simulink model "LKAS_AutoSave_DF_20220315_0945"  (R2018b)
settings: Solver=FixedStepDiscrete  StartTime=0.0  StopTime=10.0  FixedStep=0.01  RelTol=1e-3
InitFcn:
  | tmpVer = ver('MATLAB');
  | tmpVer = str2num(tmpVer.Version);
  | % -------------------------------------------------------------------
  | %  MATLAB file generated by Simulink.saveVars on 21-Nov-2019 10:06:14
  | %  MATLAB version: 7.13.0.564 (R2011b)
  | % -------------------------------------------------------------------
  | 
  | 
  | SInt16 = Simulink.AliasType;
  | SInt16.Description = 'Num';
  | if (tmpVer > 7.11)
  | 	SInt16.DataScope = 'Auto';
  | end
  | SInt16.HeaderFile = 'Rte_Type.h';
  | SInt16.BaseType = 'int16';
  | 
  | SInt32 = Simulink.AliasType;
  | SInt32.Description = 'Num';
  | if (tmpVer > 7.11)
  | 	SInt32.DataScope = 'Auto';
  | end
  | SInt32.HeaderFile = 'Rte_Type.h';
  | SInt32.BaseType = 'int32';
  | 
  | SInt8 = Simulink.AliasType;
  | SInt8.Description = 'Num';
  | if (tmpVer > 7.11)
  | 	SInt8.DataScope = 'Auto';
  | end
  | SInt8.HeaderFile = 'Rte_Type.h';
  | SInt8.BaseType = 'int8';
  | 
  | T_A_m2_1024_1_u32 = Simulink.NumericType;
  | T_A_m2_1024_1_u32.Description = 'm2 (square meters  (m2))';
  | if (tmpVer > 7.11)
  | 	T_A_m2_1024_1_u32.DataScope = 'Auto';
  | end
  | T_A_m2_1024_1_u32.HeaderFile = 'Rte_Type.h';
  | T_A_m2_1024_1_u32.DataTypeMode = 'Fixed-point: slope and bias scaling';
  | T_A_m2_1024_1_u32.SignednessBool = false;
  | T_A_m2_1024_1_u32.WordLength = 32;
  | T_A_m2_1024_1_u32.FixedExponent = -10;
  | T_A_m2_1024_1_u32.SlopeAdjustmentFactor = 1;
  | T_A_m2_1024_1_u32.Bias = 0;
  | T_A_m2_1024_1_u32.DataTypeOverride = 'Inherit';
  | T_A_m2_1024_1_u32.IsAlias = true;
  | 
  | T_A_m2_65536_1_u16 = Simulink.NumericType;
  | T_A_m2_65536_1_u16.Description = 'm2 (square meters  (m2))';
  | if (tmpVer > 7.11)
  | 	T_A_m2_65536_1_u16.DataScope = 'Auto';
  | end
  | T_A_m2_65536_1_u16.HeaderFile = 'Rte_Type.h';
  | T_A_m2_65536_1_u16.DataTypeMode = 'Fixed-point: slope and bias scaling';
  | T_A_m2_65536_1_u16.SignednessBool = false;
  | T_A_m2_65536_1_u16.WordLength = 16;
  | T_A_m2_65536_1_u16.FixedExponent = -16;
  | T_A_m2_65536_1_u16.SlopeAdjustmentFactor = 1;
  | T_A_m2_65536_1_u16.Bias = 0;
  | T_A_m2_65536_1_u16.DataTypeOverride = 'Inherit';
  | ... (+4647 lines)
StopFcn:
  | clear  T_A_m2_1024_1_u32 T_A_m2_65536_1_u16 T_A_m2_Float32 T_A_mm2_10_1_u16 T_A_mm2_4_1_s16 T_A_mm2_Float32 T_Cnt_Num_10_1_u32 T_Cnt_Num_1_1_s16 T_Cnt_Num_1_1_s32 T_Cnt_Num_1_1_s8 T_Cnt_Num_1_1_u16 T_Cnt_Num_1_1_u32 T_Cnt_Num_1_1_u8 T_E_J_1_1_s32 T_E_J_Float32 T_E_kJ_128_1_s32 T_E_kJ_Float32 T_E_kwh_10_1_u16 T_E_kwh_Float32 T_Epl_kwhpkm_100_1_u16 T_Epl_kwhpkm_Float32 T_F_N_1_1_s16 T_F_N_Float32 T_I_A_1000_1_u16 T_I_A_1048576_1_s32 T_I_A_2048_1_s16 T_I_A_32_1_s16 T_I_A_Float32 T_I_mA_1_1_s16 T_I_mA_32768_128_s16 T_I_mA_Float32 T_J_kgpm2_128_1_u16 T_J_kgpm2_Float32 T_K_NA_1000_1_s16 T_K_NA_100_1_s16 T_K_NA_100_1_u16 T_K_NA_1024_1_s16 T_K_NA_1024_1_u16 T_K_NA_128_1_s16 T_K_NA_128_1_u16 T_K_NA_128_1_u8 T_K_NA_16777216_1_u32 T_K_NA_16_1_s16 T_K_NA_16_1_u16 T_K_NA_16_1_u8 T_K_NA_1_16_u16 T_K_NA_1_1_s16 T_K_NA_1_1_u16 T_K_NA_1_1_u8 T_K_NA_32768_1_s16 T_K_NA_32768_1_u16 T_K_NA_32_1_s8 T_K_NA_4096_1_u16 T_K_NA_4194304_1_s32 T_K_NA_4194304_1_u16 T_K_NA_65536_1_s32 T_K_NA_65536_1_u16 T_K_NA_8192_1_s16 T_K_NA_8_1_s16 T_K_NA_Float32 T_M_Nm_16_1_s16 T_M_Nm_1_1_s16 T_M_Nm_32768_1_s16 T_M_Nm_32_1_s16 T_M_Nm_4_1_s16 T_M_Nm_512_1_s16 T_M_Nm_Float32 T_P_W_1_4_s16 T_P_W_1_8_s16 T_P_W_Float32 T_P_kW_128_1_s16 T_P_kW_1_8_s16 T_P_kW_8_1_s32 T_P_kW_Float32 T_Pct_pct_1024_1_s32 T_Pct_pct_1024_1_u32 T_Pct_pct_10_1_s16 T_Pct_pct_10_1_u32 T_Pct_pct_128_100_s8 T_Pct_pct_1_1_s16 T_Pct_pct_1_4_u8 T_Pct_pct_255_100_u16 T_Pct_pct_255_100_u8 T_Pct_pct_256_1_s16 T_Pct_pct_256_1_u16 T_Pct_pct_65535_100_u16 T_Pct_pct_Float32 T_R_ohm_1024_1_s16 T_R_ohm_32_1_s16 T_R_ohm_Float32 T_TK_K_16_1_s16 T_TK_K_Float32 T_T_degC_10_400_1_u16 T_T_degC_16_1_s16 T_T_degC_1_40_1_u8 T_T_degC_2_80_1_u8 T_T_degC_Float32 T_U_V_1000_1_u16 T_U_V_10_1_u8 T_U_V_200_1_u8 T_U_V_32_1_s16 T_U_V_4096_1_s16 T_U_V_512_1_s16 T_U_V_65535_8_u16 T_U_V_8192_1_u16 T_U_V_Float32 T_U_mV_1_1_s16 T_U_mV_256_20_u16 T_U_mV_Float32 T_V_l_256_1_s16 T_V_l_4096_1_s16 T_V_l_64_1_s16 T_V_l_65535_100_u16 T_V_l_Float32 T_V_ml_128_1_s16 T_V_ml_1_1_s16 T_V_ml_32768_1_s16 T_V_ml_Float32 T_V_ul_32_1_u16 T_V_ul_Float32 T_Vpl_clpkm_512_1_u16 T_Vpl_clpkm_Float32 T_a_kphps_16_1_s16 T_a_kphps_Float32 T_a_mps2_128_1_s16 T_a_mps2_Float32 T_c_MJpkg_256_1_s16 T_c_MJpkg_Float32 T_c_kJpgpK_1024_1_s16 T_c_kJpgpK_Float32 T_c_kJpkgpK_128_1_u16 T_c_kJpkgpK_Float32 T_chrg_Ah_1_1_s16 T_chrg_Ah_1_1_u16 T_chrg_Ah_1_1_u8 T_chrg_Ah_256_1_u16 T_chrg_Ah_4194304_1_s32 T_chrg_Ah_512_1_u16 T_chrg_Ah_8_1_u16 T_chrg_Ah_Float32 T_cmp_NA_100_1_s16 T_cmp_NA_128_1_s16 T_cmp_NA_16_1_s16 T_cmp_NA_32768_1_u16 T_cmp_NA_Float32 T_d2n_rpmps2_4_1_s16 T_d2n_rpmps2_Float32 T_dPct_pctps_16_1_s16 T_dPct_pctps_256_1_s16 T_dPct_pctps_Float32 T_dT_degCps_128_1_s16 T_dT_degCps_Float32 T_dV_lph_1_1_s16 T_dV_lph_Float32 T_dV_lpm_128_1_s16 T_dV_lpm_32_1_s16 T_dV_lpm_Float32 T_dV_lps_1024_1_u16 T_dV_lps_4_1_u16 T_dV_lps_Float32 T_dV_mlps_1024_1_s16 T_dV_mlps_Float32 T_d_BitField16 T_dm_gps_128_1_s16 T_dm_gps_128_1_u16 T_dm_gps_256_1_u16 T_dm_gps_Float32 T_dm_mgps_1_1_s16 T_dm_mgps_Float32 T_dn_rpmps_1_1_s16 T_dn_rpmps_2_1_s16 T_dn_rpmps_Float32 T_dp_Paps_1_1_s16 T_dp_Paps_Float32 T_dp_kPaps_1_1_s16 T_dp_kPaps_8_1_s16 T_dp_kPaps_Float32 T_dphi_degps_128_1_s16 T_dphi_degps_8_1_s16 T_dphi_degps_Float32 T_dr_ps_256_1_s16 T_dr_ps_Float32 T_drho_mgplps_1_2_s16 T_drho_mgplps_Float32 T_e_NA_1_1_u8 T_f_Hz_1_1_u16 T_f_Hz_1_1_u32 T_f_Hz_64_1_u16 T_f_Hz_8_1_s16 T_f_Hz_Float32 T_g_BitField32 T_l_km_16_1_s16 T_l_km_1_1_u16 T_l_km_1_1_u32 T_l_km_Float32 T_l_m_1024_1_s16 T_l_m_16_1_s16 T_l_m_1_1_u32 T_l_m_Float32 T_l_mm_16_1_s16 T_l_mm_1_1_u16 T_l_mm_4096_1_s16 T_l_mm_4_1_u8 T_l_mm_64_1_s16 T_l_mm_Float32 T_m_g_1_1_s16 T_m_g_2048_1_s16 T_m_g_32_1_u16 T_m_g_Float32 T_m_kg_1024_1_s16 T_m_kg_1_1_s16 T_m_kg_1_1_u32 T_m_kg_Float32 T_m_mg_128_1_s16 T_m_mg_32_1_s16 T_m_mg_Float32 T_n_rpm_1_1_s16 T_n_rpm_1_25_u8 T_n_rpm_256_50_u16 T_n_rpm_2_25_u8 T_n_rpm_4_1_u16 T_n_rpm_Float32 T_p_MPa_64_1_s16 T_p_MPa_Float32 T_p_Pa_1_1_s16 T_p_Pa_Float32 T_p_kPa_1_10_u16 T_p_kPa_1_1_s16 T_p_kPa_1_1_u8 T_p_kPa_256_1_u16 T_p_kPa_32_1_u16 T_p_kPa_64_1_s16 T_p_kPa_Float32 T_phi_deg_100_1_s16 T_phi_deg_1024_1_s16 T_phi_deg_128_1_s16 T_phi_deg_1_1_u8 T_phi_deg_256_1_s16 T_phi_deg_2_1_s8 T_phi_deg_32_1_s16 T_phi_deg_512_6_s32 T_phi_deg_Float32 T_phi_rad_2048_1_s16 T_phi_rad_Float32 T_r_NA_1024_1_s16 T_r_NA_1024_1_u16 T_r_NA_16384_1_s16 T_r_NA_16_1_s16 T_r_NA_256_1_s8 T_r_NA_256_1_u16 T_r_NA_32768_1_u16 T_r_NA_32_1_u16 T_r_NA_4096_1_s16 T_r_NA_65535_2_u16 T_r_NA_8192_1_u16 T_r_NA_Float32 T_rho_gpl_8192_1_s16 T_rho_gpl_Float32 T_rho_kgpm3_16_1_s16 T_rho_kgpm3_Float32 T_rho_mgpl_1_1_s16 T_rho_mgpl_64_1_s16 T_rho_mgpl_Float32 T_t_hour_1_1_s16 T_t_hour_Float32 T_t_m_1_1_u16 T_t_m_Float32 T_t_ms_1_1_s16 T_t_ms_1_1_u16 T_t_ms_1_1_u32 T_t_ms_4096_1_s16 T_t_ms_64_1_s16 T_t_ms_Float32 T_t_s_1000_1_s16 T_t_s_100_1_s16 T_t_s_10_1_s16 T_t_s_10_1_u16 T_t_s_1_1_s16 T_t_s_1_1_u16 T_t_s_1_1_u32 T_t_s_Float32 T_t_us_10_1_u32 T_t_us_1_1_s16 T_t_us_1_1_u32 T_t_us_1_4_u16 T_t_us_Float32 T_v_kph_1_1_u8 T_v_kph_64_1_s16 T_v_kph_64_1_u16 T_v_kph_Float32 T_v_mps_256_1_s16 T_v_mps_Float32 T_w_radps_32_1_s16 T_w_radps_Float32 T_y_BitField8 T_y_BitFieldDiagProgress T_y_BitFieldDiagStatus T_y_NA_1_1_u8 SInt16 SInt32 SInt8 T_BOOLEAN UInt16 UInt32 UInt8 s16 s32 s8 u16 u32 u8
model workspace (MAT data in the model file):
  MCOS : class17 (value not decoded)
  MCOS : class17 (value not decoded)
  MCOS : class17 (value not decoded)
  MCOS : class17 (value not decoded)
  MCOS : class17 (value not decoded)
  MCOS : class17 (value not decoded)
  MCOS : class17 (value not decoded)
  MCOS : class17 (value not decoded)
  MCOS : class17 (value not decoded)
  MCOS : class17 (value not decoded)
  MCOS : class17 (value not decoded)
  MCOS : class17 (value not decoded)
  MCOS : class17 (value not decoded)
  MCOS : class17 (value not decoded)
  MCOS : class17 (value not decoded)
  MCOS : class17 (value not decoded)
  MCOS : class17 (value not decoded)
  MCOS : class17 (value not decoded)
  MCOS : class17 (value not decoded)
  MCOS : class17 (value not decoded)
  MCOS : class17 (value not decoded)
  MCOS : class17 (value not decoded)
  MCOS : class17 (value not decoded)
  MCOS : class17 (value not decoded)
  MCOS : class17 (value not decoded)
  MCOS : class17 (value not decoded)
  MCOS : class17 (value not decoded)
  MCOS : class17 (value not decoded)
  MCOS : class17 (value not decoded)
  MCOS : class17 (value not decoded)
  MCOS : class17 (value not decoded)
  MCOS : class17 (value not decoded)
  MCOS : class17 (value not decoded)
  MCOS : class17 (value not decoded)
  MCOS : class17 (value not decoded)
  MCOS : class17 (value not decoded)
  MCOS : class17 (value not decoded)
  MCOS : class17 (value not decoded)
  MCOS : class17 (value not decoded)
  MCOS : class17 (value not decoded)
  MCOS : class17 (value not decoded)
  MCOS : class17 (value not decoded)
  MCOS : class17 (value not decoded)
  MCOS : class17 (value not decoded)
  MCOS : class17 (value not decoded)
  MCOS : class17 (value not decoded)
  MCOS : class17 (value not decoded)
  MCOS : class17 (value not decoded)
  MCOS : class17 (value not decoded)
  MCOS : class17 (value not decoded)
  MCOS : class17 (value not decoded)
  MCOS : class17 (value not decoded)
  MCOS : class17 (value not decoded)
  MCOS : class17 (value not decoded)
  MCOS : class17 (value not decoded)
  MCOS : class17 (value not decoded)
  MCOS : class17 (value not decoded)
  MCOS : class17 (value not decoded)
  MCOS : class17 (value not decoded)
  MCOS : class17 (value not decoded)
  MCOS : class17 (value not decoded)
  MCOS : class17 (value not decoded)
  MCOS : class17 (value not decoded)
  MCOS : class17 (value not decoded)
  MCOS : class17 (value not decoded)
  MCOS : class17 (value not decoded)
  MCOS : class17 (value not decoded)
  MCOS : class17 (value not decoded)
  MCOS : class17 (value not decoded)
  MCOS : class17 (value not decoded)
  MCOS : class17 (value not decoded)
  MCOS : class17 (value not decoded)
  MCOS : class17 (value not decoded)
  MCOS : class17 (value not decoded)
  MCOS : class17 (value not decoded)
  MCOS : class17 (value not decoded)
  MCOS : class17 (value not decoded)
  MCOS : class17 (value not decoded)
  MCOS : class17 (value not decoded)
  MCOS : class17 (value not decoded)
  MCOS : class17 (value not decoded)
  MCOS : class17 (value not decoded)
  MCOS : class17 (value not decoded)
  MCOS : class17 (value not decoded)
  MCOS : class17 (value not decoded)
  MCOS : class17 (value not decoded)
  MCOS : class17 (value not decoded)
  MCOS : class17 (value not decoded)
  MCOS : class17 (value not decoded)
  MCOS : class17 (value not decoded)
  MCOS : class17 (value not decoded)
  MCOS : class17 (value not decoded)
  MCOS : class17 (value not decoded)
  MCOS : class17 (value not decoded)
  MCOS : class17 (value not decoded)
  MCOS : class17 (value not decoded)
  MCOS : class17 (value not decoded)
  MCOS : class17 (value not decoded)
  MCOS : class17 (value not decoded)
  MCOS : class17 (value not decoded)
  MCOS : class17 (value not decoded)
  MCOS : class17 (value not decoded)
  MCOS : class17 (value not decoded)
  MCOS : class17 (value not decoded)
undefined symbols (not defined in the file): LKA_CarWidth, LKA_SampleTime, LKA_StrRatio_C, LKA_Veh2CamL_C, LKA_Veh2CamW_C, LKA_WhlBaseL_C, LL_CompHdAg_C, LL_CompSWA_C, LL_CrvtPrvwT_C, LL_DesDvt_C, LL_DvtComp_C, LL_DvtPrvwT_C, LL_DvtSpdDet_vDvtSpdMin_C, LL_HandsOff_ExitTime, LL_HandsOff_TextTime, LL_HandsOff_WarnTime, LL_HdAgExT_C, LL_HdAgPrvwT_C, LL_LAccMax_C, LL_LAccRMax_C, LL_LDW_EarliestWarnLine_C, LL_LDW_LatestWarnLine_C, LL_LDWS_SUPPRESS_HEADING, LL_LFClb_TFC_FfCtlRatio_C, LL_LFClb_TFC_KdBalance_C, LL_LFClb_TFC_KdMaxSWA_C, LL_LFClb_TFC_KdV1_C, LL_LFClb_TFC_KdV2_C, LL_LFClb_TFC_KdVehSpdLwr_C, LL_LFClb_TFC_KdVehSpdUpr_C, LL_LFClb_TFC_Ki_C, LL_LFClb_TFC_KiMaxSWA_C, LL_LFClb_TFC_Kp_C, LL_LFClb_TFC_KpKlat_C, LL_LFClb_TFC_KpV1_C, LL_LFClb_TFC_KpV2_C, LL_LFClb_TFC_KpVehSpdLwr_C, LL_LFClb_TFC_KpVehSpdUpr_C, LL_LFClb_TFC_PrvwT_C, LL_LKA_EarliestWarnLine_C, LL_LKA_LatestWarnLine_C, LL_LKAExPrcs_ExitC0Dvt, LL_LKAExPrcs_ExitC0Swt, LL_LKAExPrcs_tiExitDelayTime3, LL_LKAExPrcs_tiExitTime1, LL_LKAExPrcs_tiExitTime2, LL_LKAExPrcs_tiExitTime3, LL_LKAS_OUT_OF_CONTROL_LAT_VEL, LL_LKAS_OUT_OF_CONTROL_TTLC, LL_LKASWASyn_M0, LL_LKASWASyn_M1, LL_LKASWASyn_M2, LL_LKASWASyn_M3D, LL_LKASWASyn_M3K, LL_LKASWASyn_SWAaddMax, LL_LKASWASyn_T2, LL_LKASWASyn_tiTrqSwaRtTime, LL_LKASWASyn_tiTrqSwaTime, LL_LKASWASyn_TrqMax, LL_LKASWASyn_TrqSwaAddSwt ... (+45)
libraries: simulink x139, canmsglib x8, dspstat3 x3, simulink_extras x1
(part 18 of 20)

== system LKAS_AutoSave_DF_20220315_0945/LKAS/LL/LLOn/LL State Determination (LLStateDet)/LL State Machine Conditions (LLSMCon)/Deactivation Condition (DeactvC)/Deviation Threshold Condition (DvtThresCon)/Deviation Threshold Judgement LDW (DvtThresJdg)/Deviation Threshold Condition Synthesis (DTCSyn) ==
  note: 累计激活LDW的时间，报警时间超过2s触发Deactive;
      | 检测到上升沿，即从离开报警区域，到再次进入报警区域，触发Activeflg，重新计时。
  DTCSyn_stLftDvtThresActvFlg : Inport
  DTCSyn_stRgtDvtThresActvFlg : Inport  Port=2
  DTCSyn_stDvtSpdFlg : Inport  Port=3
  SampleTime : Inport  Port=4
  Bus Selector1 : BusSelector  OutputSignals=bsConstantClb.LKA_SampleTime
  Cast To Single{,1,3..4} (4 alike) : DataTypeConversion  OutDataTypeStr=uint8
  Cast To Single2 : DataTypeConversion  LockScale=on
  Constant : Constant  Value=2  OutDataTypeStr=single
  Constant2 : Constant  Value=0  OutDataTypeStr=uint8
  Divide : Product  Inputs=**  OutDataTypeStr=uint8
  Gain1 : Gain  Gain=2  OutDataTypeStr=Inherit: Same as input
  Sum Condition : Subsystem
  Switch2 : Switch  Criteria=u2 > Threshold
  Switch3 : Switch
  DTCSyn_stDvtThresActvFlg : Outport
  wires:
  Cast To Single1/1 -> Gain1/1
  Cast To Single/1 -> Cast To Single2/1
  Gain1/1 -> Switch3/3  "DvtThresActvFlg"
  Cast To Single2/1 -> Switch2/1  "DvtThresActvFlg"
  Constant2/1 -> Switch2/3  "DvtThresActvFlg"
  DTCSyn_stDvtSpdFlg/1 -> Switch2/2, Switch3/2
  Switch2/1 -> Switch3/1
  DTCSyn_stLftDvtThresActvFlg/1 -> Cast To Single/1
  DTCSyn_stRgtDvtThresActvFlg/1 -> Cast To Single1/1
  Bus Selector1/1 -> Sum Condition/1(In)  "<LKA_SampleTime>"
  Constant/1 -> Sum Condition/2(Sum)
  SampleTime/1 -> Bus Selector1/1
  Switch3/1 -> Cast To Single3/1, Sum Condition/Enable
  Sum Condition/1(Out) -> Cast To Single4/1
  Divide/1 -> DTCSyn_stDvtThresActvFlg/1
  Cast To Single3/1 -> Divide/1
  Cast To Single4/1 -> Divide/2

== system LKAS_AutoSave_DF_20220315_0945/LKAS/LL/LLOn/LL State Determination (LLStateDet)/LL State Machine Conditions (LLSMCon)/Deactivation Condition (DeactvC)/Deviation Threshold Condition (DvtThresCon)/Deviation Threshold Judgement LDW (DvtThresJdg)/Left Side Deviation Threshold Condition (LftDTC) ==
  LftDTC_bsDvtThresInfo : Inport
  LftDTC_lLftDvt : Inport  Port=2
  LftDTC_vLftDvtSpd : Inport  Port=3
  Abs : Abs
  Bus Selector : BusSelector  OutputSignals=LL_ThresDet_lDvtThresLwrLDW,LL_ThresDet_lDvtThresUprLDW,LL_ThresDet_tiTTLCThresLDW
  Divide : Product  Inputs=**
  Relational Operator2 : RelationalOperator  Operator=<=  OutDataTypeStr=boolean  RndMeth=Nearest
  Saturation Dynamic : simulink/Discontinuities/Saturation Dynamic  OutMin=[]  OutMax=[]  OutDataTypeStr=Inherit: Same as second input  OutDataType=fixdt(1, 16)  OutScaling=2^-10  DoSatur=off
  LftDTC_stLftDvtThresActvFlg : Outport
  wires:
  Abs/1 -> Divide/2
  Saturation Dynamic/1 -> Relational Operator2/2
  Divide/1 -> Saturation Dynamic/2
  LftDTC_vLftDvtSpd/1 -> Abs/1
  LftDTC_lLftDvt/1 -> Relational Operator2/1
  Relational Operator2/1 -> LftDTC_stLftDvtThresActvFlg/1
  Bus Selector/2 -> Saturation Dynamic/1  "<LL_ThresDet_lDvtThresUprLDW>"
  Bus Selector/3 -> Divide/1  "<LL_ThresDet_tiTTLCThresLDW>"
  Bus Selector/1 -> Saturation Dynamic/3  "<LL_ThresDet_lDvtThresLwrLDW>"
  LftDTC_bsDvtThresInfo/1 -> Bus Selector/1

== system LKAS_AutoSave_DF_20220315_0945/LKAS/LL/LLOn/LL State Determination (LLStateDet)/LL State Machine Conditions (LLSMCon)/Deactivation Condition (DeactvC)/Deviation Threshold Condition (DvtThresCon)/Deviation Threshold Judgement LDW (DvtThresJdg)/Right Side Deviation Threshold Condition (RgtDTC) ==
  RgtDTC_bsDvtThresInfo : Inport
  RgtDTC_lRgtDvt : Inport  Port=2
  RgtDTC_vRgtDvtSpd : Inport  Port=3
  Abs : Abs
  Bus Selector : BusSelector  OutputSignals=LL_ThresDet_lDvtThresLwrLDW,LL_ThresDet_lDvtThresUprLDW,LL_ThresDet_tiTTLCThresLDW
  Divide : Product  Inputs=**
  Relational Operator2 : RelationalOperator  Operator=<=  OutDataTypeStr=boolean  RndMeth=Nearest
  Saturation Dynamic : simulink/Discontinuities/Saturation Dynamic  OutMin=[]  OutMax=[]  OutDataTypeStr=Inherit: Same as second input  OutDataType=fixdt(1, 16)  OutScaling=2^-10  DoSatur=off
  RgtDTC_stRgtDvtThresActvFlg : Outport
  wires:
  Bus Selector/3 -> Divide/1  "<LL_ThresDet_tiTTLCThresLDW>"
  Bus Selector/2 -> Saturation Dynamic/1  "<LL_ThresDet_lDvtThresUprLDW>"
  Bus Selector/1 -> Saturation Dynamic/3  "<LL_ThresDet_lDvtThresLwrLDW>"
  RgtDTC_vRgtDvtSpd/1 -> Abs/1
  Saturation Dynamic/1 -> Relational Operator2/2
  Divide/1 -> Saturation Dynamic/2
  Abs/1 -> Divide/2
  RgtDTC_lRgtDvt/1 -> Relational Operator2/1
  Relational Operator2/1 -> RgtDTC_stRgtDvtThresActvFlg/1
  RgtDTC_bsDvtThresInfo/1 -> Bus Selector/1

== system LKAS_AutoSave_DF_20220315_0945/LKAS/LL/LLOn/LL State Determination (LLStateDet)/LL State Machine Conditions (LLSMCon)/Deactivation Condition (DeactvC)/Deviation Threshold Condition (DvtThresCon)/Deviation Threshold Judgement LKA (DvtThresJdg)/Deviation Speed Detection (DvtSpdDet) ==
  DvtSpdDet_vLftDvtSpd : Inport
  DvtSpdDet_vRgtDvtSpd : Inport  Port=2
  DvtSpdDet_vDvtSpdMin_C : Inport  Port=3
  If : If  NumInputs=3  IfExpression=u1>=u3 | u2>=u3  ElseIfExpressions=u1<=-u3 | u2<=-u3
  Merge1 : Merge  Inputs=3
  Ph1SWA : Subsystem
  Ph2SWA : Subsystem
  Ph3SWA : Subsystem
  DvtSpdDet_stDvtSpdFlg : Outport
  wires:
  DvtSpdDet_vLftDvtSpd/1 -> If/1
  DvtSpdDet_vRgtDvtSpd/1 -> If/2
  DvtSpdDet_vDvtSpdMin_C/1 -> If/3
  If/1 -> Ph1SWA/Action
  Ph1SWA/1(Out) -> Merge1/1
  Ph2SWA/1(Out) -> Merge1/2
  Ph3SWA/1(Out) -> Merge1/3
  If/2 -> Ph2SWA/Action
  If/3 -> Ph3SWA/Action
  Merge1/1 -> DvtSpdDet_stDvtSpdFlg/1

== system LKAS_AutoSave_DF_20220315_0945/LKAS/LL/LLOn/LL State Determination (LLStateDet)/LL State Machine Conditions (LLSMCon)/Deactivation Condition (DeactvC)/Deviation Threshold Condition (DvtThresCon)/Deviation Threshold Judgement LKA (DvtThresJdg)/Deviation Threshold Condition Synthesis (DTCSyn) ==
  DTCSyn_stLftDvtThresActvFlg : Inport
  DTCSyn_stRgtDvtThresActvFlg : Inport  Port=2
  DTCSyn_stDvtSpdFlg : Inport  Port=3
  Cast To Single : DataTypeConversion  OutDataTypeStr=uint8
  Cast To Single1 : DataTypeConversion  OutDataTypeStr=uint8
  Cast To Single2 : DataTypeConversion  LockScale=on
  Constant2 : Constant  Value=0  OutDataTypeStr=uint8
  Gain1 : Gain  Gain=2  OutDataTypeStr=Inherit: Same as input
  Switch2 : Switch  Criteria=u2 > Threshold
  Switch3 : Switch
  DTCSyn_stDvtThresActvFlg : Outport
  wires:
  Cast To Single1/1 -> Gain1/1
  Cast To Single/1 -> Cast To Single2/1
  Switch2/1 -> Switch3/1
  Switch3/1 -> DTCSyn_stDvtThresActvFlg/1
  Constant2/1 -> Switch2/3  "DvtThresActvFlg"
  DTCSyn_stDvtSpdFlg/1 -> Switch2/2, Switch3/2
  Cast To Single2/1 -> Switch2/1  "DvtThresActvFlg"
  Gain1/1 -> Switch3/3  "DvtThresActvFlg"
  DTCSyn_stLftDvtThresActvFlg/1 -> Cast To Single/1
  DTCSyn_stRgtDvtThresActvFlg/1 -> Cast To Single1/1

== system LKAS_AutoSave_DF_20220315_0945/LKAS/LL/LLOn/LL State Determination (LLStateDet)/LL State Machine Conditions (LLSMCon)/Deactivation Condition (DeactvC)/Deviation Threshold Condition (DvtThresCon)/Deviation Threshold Judgement LKA (DvtThresJdg)/Left Side Deviation Threshold Condition (LftDTC) ==
  LftDTC_bsDvtThresInfo : Inport
  LftDTC_lLftDvt : Inport  Port=2
  LftDTC_vLftDvtSpd : Inport  Port=3
  Abs : Abs
  Bus Selector : BusSelector  OutputSignals=LL_ThresDet_lDvtThresLwrLKA,LL_ThresDet_lDvtThresUprLKA,LL_ThresDet_tiTTLCThresLKA
  Constant : Constant  Value=0  OutDataTypeStr=single
  Divide : Product  Inputs=**
  Logical Operator : Logic  AllPortsSameDT=off  OutDataTypeStr=boolean
  Relational Operator1 : RelationalOperator  Operator=<  OutDataTypeStr=boolean  RndMeth=Nearest
  Relational Operator3 : RelationalOperator  Operator=<=  OutDataTypeStr=boolean  RndMeth=Nearest
  Saturation Dynamic : simulink/Discontinuities/Saturation Dynamic  OutMin=[]  OutMax=[]  OutDataTypeStr=Inherit: Same as second input  OutDataType=fixdt(1, 16)  OutScaling=2^-10  DoSatur=off
  LftDTC_stLftDvtThresActvFlg : Outport
  wires:
  LftDTC_bsDvtThresInfo/1 -> Bus Selector/1
  Bus Selector/1 -> Saturation Dynamic/3  "<LL_ThresDet_lDvtThresLwrLKA>"
  Bus Selector/3 -> Divide/1  "<LL_ThresDet_tiTTLCThresLKA>"
  Bus Selector/2 -> Saturation Dynamic/1  "<LL_ThresDet_lDvtThresUprLKA>"
  Relational Operator3/1 -> Logical Operator/2
  LftDTC_lLftDvt/1 -> Relational Operator1/2, Relational Operator3/1
  LftDTC_vLftDvtSpd/1 -> Abs/1
  Divide/1 -> Saturation Dynamic/2
  Saturation Dynamic/1 -> Relational Operator3/2
  Abs/1 -> Divide/2
  Logical Operator/1 -> LftDTC_stLftDvtThresActvFlg/1
  Constant/1 -> Relational Operator1/1
  Relational Operator1/1 -> Logical Operator/1

== system LKAS_AutoSave_DF_20220315_0945/LKAS/LL/LLOn/LL State Determination (LLStateDet)/LL State Machine Conditions (LLSMCon)/Deactivation Condition (DeactvC)/Deviation Threshold Condition (DvtThresCon)/Deviation Threshold Judgement LKA (DvtThresJdg)/Right Side Deviation Threshold Condition (RgtDTC) ==
  RgtDTC_bsDvtThresInfo : Inport
  RgtDTC_lRgtDvt : Inport  Port=2
  RgtDTC_vRgtDvtSpd : Inport  Port=3
  Abs : Abs
  Bus Selector : BusSelector  OutputSignals=LL_ThresDet_lDvtThresLwrLKA,LL_ThresDet_lDvtThresUprLKA,LL_ThresDet_tiTTLCThresLKA
  Constant : Constant  Value=0  OutDataTypeStr=single
  Divide : Product  Inputs=**
  Logical Operator : Logic  AllPortsSameDT=off  OutDataTypeStr=boolean
  Relational Operator1 : RelationalOperator  Operator=<  OutDataTypeStr=boolean  RndMeth=Nearest
  Relational Operator2 : RelationalOperator  Operator=<=  OutDataTypeStr=boolean  RndMeth=Nearest
  Saturation Dynamic : simulink/Discontinuities/Saturation Dynamic  OutMin=[]  OutMax=[]  OutDataTypeStr=Inherit: Same as second input  OutDataType=fixdt(1, 16)  OutScaling=2^-10  DoSatur=off
  RgtDTC_stRgtDvtThresActvFlg : Outport
  wires:
  Abs/1 -> Divide/2
  RgtDTC_bsDvtThresInfo/1 -> Bus Selector/1
  Relational Operator2/1 -> Logical Operator/2
  RgtDTC_vRgtDvtSpd/1 -> Abs/1
  Divide/1 -> Saturation Dynamic/2
  Saturation Dynamic/1 -> Relational Operator2/2
  Bus Selector/1 -> Saturation Dynamic/3  "<LL_ThresDet_lDvtThresLwrLKA>"
  Bus Selector/2 -> Saturation Dynamic/1  "<LL_ThresDet_lDvtThresUprLKA>"
  Bus Selector/3 -> Divide/1  "<LL_ThresDet_tiTTLCThresLKA>"
  Constant/1 -> Relational Operator1/1
  Relational Operator1/1 -> Logical Operator/1
  RgtDTC_lRgtDvt/1 -> Relational Operator1/2, Relational Operator2/1
  Logical Operator/1 -> RgtDTC_stRgtDvtThresActvFlg/1

== system LKAS_AutoSave_DF_20220315_0945/LKAS/LL/LLOn/LL State Determination (LLStateDet)/LL State Machine Conditions (LLSMCon)/Deactivation Condition (DeactvC)/Driver Take Condition (DvrTkCon)/Time Delay (TDel)/If Action Subsystem ==
  Action Port : ActionPort  InitializeStates=reset  ActionType=then
      settings: AttributesFormatString=states = %<InitializeStates>
  Constant : Constant  OutDataTypeStr=boolean  SampleTime=-1
  Out : Outport
      settings: AttributesFormatString=%<OutputWhenDisabled> = %<InitialOutput>
  wires:
  Constant/1 -> Out/1

== system LKAS_AutoSave_DF_20220315_0945/LKAS/LL/LLOn/LL State Determination (LLStateDet)/LL State Machine Conditions (LLSMCon)/Deactivation Condition (DeactvC)/Driver Take Condition (DvrTkCon)/Time Delay (TDel)/If Action Subsystem1 ==
  Action Port : ActionPort  InitializeStates=reset  ActionType=elseif
      settings: AttributesFormatString=states = %<InitializeStates>
  Constant : Constant  Value=0  OutDataTypeStr=boolean  SampleTime=-1
  Out : Outport
      settings: AttributesFormatString=%<OutputWhenDisabled> = %<InitialOutput>
  wires:
  Constant/1 -> Out/1

== system LKAS_AutoSave_DF_20220315_0945/LKAS/LL/LLOn/LL State Determination (LLStateDet)/LL State Machine Conditions (LLSMCon)/Deactivation Condition (DeactvC)/Driver Take Condition (DvrTkCon)/Time Delay (TDel)/If Action Subsystem3 ==
  In1 : Inport
  Action Port : ActionPort  InitializeStates=reset  ActionType=else
      settings: AttributesFormatString=states = %<InitializeStates>
  Out : Outport
      settings: AttributesFormatString=%<OutputWhenDisabled> = %<InitialOutput>
  wires:
  In1/1 -> Out/1

== system LKAS_AutoSave_DF_20220315_0945/LKAS/LL/LLOn/LL State Determination (LLStateDet)/LL State Machine Conditions (LLSMCon)/Deactivation Condition (DeactvC)/Driver Take Condition (DvrTkCon)/Time Delay (TDel)/Sum Condition1 ==
  SampleTime : Inport
  Sum : Inport  Port=2
  state = reset : EnablePort  StatesWhenEnabling=reset
  Add1 : Sum  OutDataTypeStr=single
  Memory : Memory  InheritSampleTime=on
  Relational Operator : RelationalOperator  Operator=<=  OutDataTypeStr=boolean  RndMeth=Nearest
  Saturation : Saturate  UpperLimit=5  LowerLimit=0
      settings: AttributesFormatString="Min = %<LowerLimit>  Max = %<UpperLimit>"
  Out : Outport  OutputWhenDisabled=reset  InitialOutput=0
      settings: AttributesFormatString=%<OutputWhenDisabled> = %<InitialOutput>
  wires:
  Memory/1 -> Add1/2
  Add1/1 -> Saturation/1
  SampleTime/1 -> Add1/1
  Sum/1 -> Relational Operator/2
  Relational Operator/1 -> Out/1
  Saturation/1 -> Memory/1, Relational Operator/1

== system LKAS_AutoSave_DF_20220315_0945/LKAS/LL/LLOn/LL State Determination (LLStateDet)/LL State Machine Conditions (LLSMCon)/Disable Condition (DisblC)/Driver Intent Condition (DrvInttC)/Driver Release Detection (DrvRlsDet)/ExitCount ==
  SampleTime : Inport
  ExitTime : Inport  Port=2
  Enable : EnablePort  StatesWhenEnabling=reset
  Add : Sum  OutDataTypeStr=single
  Memory : Memory  InheritSampleTime=on
  Relational Operator : RelationalOperator  OutDataTypeStr=boolean  RndMeth=Nearest
  Saturation : Saturate  UpperLimit=60  LowerLimit=0
      settings: AttributesFormatString="Min = %<LowerLimit>  Max = %<UpperLimit>"
  Out : Outport  OutputWhenDisabled=reset  InitialOutput=0
      settings: AttributesFormatString=%<OutputWhenDisabled> = %<InitialOutput>
  wires:
  Memory/1 -> Add/2
  Saturation/1 -> Relational Operator/1, Memory/1
  Add/1 -> Saturation/1
  Relational Operator/1 -> Out/1
  SampleTime/1 -> Add/1
  ExitTime/1 -> Relational Operator/2

== system LKAS_AutoSave_DF_20220315_0945/LKAS/LL/LLOn/LL State Determination (LLStateDet)/LL State Machine Conditions (LLSMCon)/Disable Condition (DisblC)/Driver Intent Condition (DrvInttC)/Take-Over Steering Check (TkOvStChk)/Sum Condition1 ==
  In : Inport
  Sum : Inport  Port=2
  state = reset : EnablePort  StatesWhenEnabling=reset
  Add1 : Sum  AccumDataTypeStr=single  OutDataTypeStr=single
  Memory : Memory  InheritSampleTime=on
  Relational Operator : RelationalOperator  OutDataTypeStr=boolean  RndMeth=Nearest
  Saturation : Saturate  UpperLimit=5000  LowerLimit=0
      settings: AttributesFormatString="Min = %<LowerLimit>  Max = %<UpperLimit>"
  Out : Outport  OutputWhenDisabled=reset  InitialOutput=0
      settings: AttributesFormatString=%<OutputWhenDisabled> = %<InitialOutput>
  wires:
  Memory/1 -> Add1/2
  Add1/1 -> Saturation/1
  In/1 -> Add1/1
  Sum/1 -> Relational Operator/2
  Relational Operator/1 -> Out/1
  Saturation/1 -> Memory/1, Relational Operator/1

== system LKAS_AutoSave_DF_20220315_0945/LKAS/LL/LLOn/LL State Determination (LLStateDet)/LL State Machine Conditions (LLSMCon)/Disable Condition (DisblC)/Driver Intent Condition (DrvInttC)/Take-Over Steering Check (TkOvStChk)/Time Delay (TDel) ==
  TDel_stFlgIn : Inport
  SampleTime : Inport  Port=2
  TDel_tiTDel : Inport  Port=3
  Detect Rise Positive : simulink/Logic and Bit Operations/Detect Rise Positive  vinit=0  OutDataTypeStr=boolean
  If : If  IfExpression=u1
  If Action Subsystem : Subsystem  TreatAsAtomicUnit=on
  If Action Subsystem3 : Subsystem  TreatAsAtomicUnit=on
  Logical Operator : Logic  Operator=OR  AllPortsSameDT=off  OutDataTypeStr=boolean
  Merge : Merge
  Sum Condition1 : Subsystem  TreatAsAtomicUnit=on
  Unit Delay : UnitDelay  SampleTime=-1
  TDel_stFlgOut : Outport
  wires:
  Logical Operator/1 -> TDel_stFlgOut/1
  SampleTime/1 -> Sum Condition1/1(SampleTime)
  If/1 -> If Action Subsystem/Action
  If/2 -> If Action Subsystem3/Action
  If Action Subsystem/1(Out) -> Merge/1
  If Action Subsystem3/1(Out) -> Merge/2
  Merge/1 -> Sum Condition1/Enable
  Unit Delay/1 -> If Action Subsystem3/1(In1)
  Sum Condition1/1(Out) -> Unit Delay/1, Logical Operator/2
  TDel_stFlgIn/1 -> Detect Rise Positive/1, Logical Operator/1
  Detect Rise Positive/1 -> If/1
  TDel_tiTDel/1 -> Sum Condition1/2(Sum)

== system LKAS_AutoSave_DF_20220315_0945/LKAS/LL/LLOn/LL State Determination (LLStateDet)/LL State Machine Conditions (LLSMCon)/Disable Condition (DisblC)/LKA Own Condition (LKAOwnC)/EPS Condition (EPSC)/If Action Subsystem ==
  Action Port : ActionPort  InitializeStates=reset  ActionType=then
      settings: AttributesFormatString=states = %<InitializeStates>
  Constant : Constant  OutDataTypeStr=boolean
  Out : Outport
      settings: AttributesFormatString=%<OutputWhenDisabled> = %<InitialOutput>
  wires:
  Constant/1 -> Out/1

== system LKAS_AutoSave_DF_20220315_0945/LKAS/LL/LLOn/LL State Determination (LLStateDet)/LL State Machine Conditions (LLSMCon)/Disable Condition (DisblC)/LKA Own Condition (LKAOwnC)/EPS Condition (EPSC)/If Action Subsystem1 ==
  Action Port : ActionPort  InitializeStates=reset  ActionType=elseif
      settings: AttributesFormatString=states = %<InitializeStates>
  Constant : Constant  OutDataTypeStr=boolean
  Out : Outport
      settings: AttributesFormatString=%<OutputWhenDisabled> = %<InitialOutput>
  wires:
  Constant/1 -> Out/1

== system LKAS_AutoSave_DF_20220315_0945/LKAS/LL/LLOn/LL State Determination (LLStateDet)/LL State Machine Conditions (LLSMCon)/Disable Condition (DisblC)/LKA Own Condition (LKAOwnC)/EPS Condition (EPSC)/If Action Subsystem3 ==
  Action Port : ActionPort  InitializeStates=reset  ActionType=else
      settings: AttributesFormatString=states = %<InitializeStates>
  Constant : Constant  Value=0  OutDataTypeStr=boolean  SampleTime=-1
  Out : Outport
      settings: AttributesFormatString=%<OutputWhenDisabled> = %<InitialOutput>
  wires:
  Constant/1 -> Out/1

== system LKAS_AutoSave_DF_20220315_0945/LKAS/LL/LLOn/LL State Determination (LLStateDet)/LL State Machine Conditions (LLSMCon)/Disable Condition (DisblC)/LKA Own Condition (LKAOwnC)/EPS Condition (EPSC)/Sum Condition1 ==
  SampleTime : Inport
  Sum : Inport  Port=2
  state = reset : EnablePort  StatesWhenEnabling=reset
  Add1 : Sum  OutDataTypeStr=single
  Memory : Memory  InheritSampleTime=on
  Relational Operator : RelationalOperator  OutDataTypeStr=boolean  RndMeth=Nearest
  Saturation : Saturate  UpperLimit=60  LowerLimit=0
      settings: AttributesFormatString="Min = %<LowerLimit>  Max = %<UpperLimit>"
  Out : Outport  OutputWhenDisabled=reset  InitialOutput=0
      settings: AttributesFormatString=%<OutputWhenDisabled> = %<InitialOutput>
  wires:
  Memory/1 -> Add1/2
  Add1/1 -> Saturation/1
  Sum/1 -> Relational Operator/2
  Relational Operator/1 -> Out/1
  Saturation/1 -> Memory/1, Relational Operator/1
  SampleTime/1 -> Add1/1

== system LKAS_AutoSave_DF_20220315_0945/LKAS/LL/LLOn/LL State Determination (LLStateDet)/LL State Machine Conditions (LLSMCon)/Enable Condition (EnaC)/LDW Own Condition (LDWOwnC)/Vehicle Position Check (VehPosChk)/Subsystem ==
  WarnLine_C : Inport
  LaneWidth : Inport  Port=2
  CarWidth : Inport  Port=3
  Constant : Constant  Value=0  OutDataTypeStr=single
  MATLAB Function : MATLAB Function  TreatAsAtomicUnit=on
  Multiply : Product
  Saturation Dynamic : simulink/Discontinuities/Saturation Dynamic  OutMin=[]  OutMax=[]  OutDataTypeStr=Inherit: Same as second input  OutDataType=fixdt(1, 16)  OutScaling=2^-10  DoSatur=off
  EnableLine : Outport
  wires:
  Constant/1 -> Saturation Dynamic/3
  Saturation Dynamic/1 -> EnableLine/1
  LaneWidth/1 -> MATLAB Function/2(LaneWidth)
  CarWidth/1 -> MATLAB Function/3(LKA_CarWidth)
  WarnLine_C/1 -> Multiply/1, Saturation Dynamic/1, MATLAB Function/1(DvtThresUprLDW)
  Multiply/1 -> Saturation Dynamic/2
  MATLAB Function/1(ThresDet_coefficient) -> Multiply/2

== system LKAS_AutoSave_DF_20220315_0945/LKAS/LL/LLOn/LL State Determination (LLStateDet)/LL State Machine Conditions (LLSMCon)/Enable Condition (EnaC)/LKA Own Condition (LKAOwnC)/Exit Lane Delay (ExLaneDel)/If Action Subsystem3 ==
  Action Port : ActionPort  InitializeStates=reset
      settings: AttributesFormatString=states = %<InitializeStates>
  Constant : Constant  OutDataTypeStr=boolean  SampleTime=-1
  Out : Outport
      settings: AttributesFormatString=%<OutputWhenDisabled> = %<InitialOutput>
  wires:
  Constant/1 -> Out/1

== system LKAS_AutoSave_DF_20220315_0945/LKAS/LL/LLOn/LL State Determination (LLStateDet)/LL State Machine Conditions (LLSMCon)/Enable Condition (EnaC)/LKA Own Condition (LKAOwnC)/Exit Lane Delay (ExLaneDel)/If Action Subsystem4 ==
  Action Port : ActionPort  InitializeStates=reset
      settings: AttributesFormatString=states = %<InitializeStates>
  Constant : Constant  Value=0  OutDataTypeStr=boolean  SampleTime=-1
  Out : Outport
      settings: AttributesFormatString=%<OutputWhenDisabled> = %<InitialOutput>
  wires:
  Constant/1 -> Out/1

== system LKAS_AutoSave_DF_20220315_0945/LKAS/LL/LLOn/LL State Determination (LLStateDet)/LL State Machine Conditions (LLSMCon)/Enable Condition (EnaC)/LKA Own Condition (LKAOwnC)/Exit Lane Delay (ExLaneDel)/If Action Subsystem5 ==
  In1 : Inport
  Action Port : ActionPort  InitializeStates=reset
      settings: AttributesFormatString=states = %<InitializeStates>
  Out : Outport
      settings: AttributesFormatString=%<OutputWhenDisabled> = %<InitialOutput>
  wires:
  In1/1 -> Out/1

== system LKAS_AutoSave_DF_20220315_0945/LKAS/LL/LLOn/LL State Determination (LLStateDet)/LL State Machine Conditions (LLSMCon)/Enable Condition (EnaC)/LKA Own Condition (LKAOwnC)/Exit Lane Delay (ExLaneDel)/Sum Condition1 ==
  In : Inport
  Sum : Inport  Port=2
  state = reset : EnablePort  StatesWhenEnabling=reset
  Add1 : Sum  OutDataTypeStr=uint16
  Memory : Memory  InheritSampleTime=on
  Relational Operator : RelationalOperator  Operator=<=  OutDataTypeStr=boolean  RndMeth=Nearest
  Saturation : Saturate  UpperLimit=60000  LowerLimit=0
      settings: AttributesFormatString="Min = %<LowerLimit>  Max = %<UpperLimit>"
  Out : Outport  OutputWhenDisabled=reset  InitialOutput=0
      settings: AttributesFormatString=%<OutputWhenDisabled> = %<InitialOutput>
  wires:
  Memory/1 -> Add1/2
  Add1/1 -> Saturation/1
  In/1 -> Add1/1
  Sum/1 -> Relational Operator/2
  Relational Operator/1 -> Out/1
  Saturation/1 -> Memory/1, Relational Operator/1

== system LKAS_AutoSave_DF_20220315_0945/LKAS/LL/LLOn/LL State Determination (LLStateDet)/LL State Machine Conditions (LLSMCon)/Enable Condition (EnaC)/LKA Own Condition (LKAOwnC)/Vehicle Position Check (VehPosChk)1/Subsystem ==
  WarnLine_C : Inport
  LaneWidth : Inport  Port=2
  VehPosChk_LKALineMax : Inport  Port=3
  VehPosChk_CarWidth : Inport  Port=4
  Constant : Constant  Value=0  OutDataTypeStr=single
  MATLAB Function : MATLAB Function  TreatAsAtomicUnit=on
  Multiply : Product
  Saturation Dynamic : simulink/Discontinuities/Saturation Dynamic  OutMin=[]  OutMax=[]  OutDataTypeStr=Inherit: Same as second input  OutDataType=fixdt(1, 16)  OutScaling=2^-10  DoSatur=off
  EnableLine : Outport
  wires:
  Constant/1 -> Saturation Dynamic/3
  Saturation Dynamic/1 -> EnableLine/1
  LaneWidth/1 -> MATLAB Function/2(LaneWidth)
  WarnLine_C/1 -> MATLAB Function/1(DvtThresUprLDW)
  VehPosChk_LKALineMax/1 -> Multiply/1, Saturation Dynamic/1
  VehPosChk_CarWidth/1 -> MATLAB Function/3(LKA_CarWidth)
  Multiply/1 -> Saturation Dynamic/2
  MATLAB Function/1(ThresDet_coefficient) -> Multiply/2

== system LKAS_AutoSave_DF_20220315_0945/LKAS/LL/LLOn/LKA/Lane Following (LF)/Trajectory Following Control (TFC)/Feedback Control (FbCtl)/Subsystem/Signal Latching2/if action  ==
  In : Inport
  Action Port : ActionPort  InitializeStates=reset  ActionType=then
  Out : Outport
  wires:
  In/1 -> Out/1

== system LKAS_AutoSave_DF_20220315_0945/LKAS/LL/LLOn/LKA/Plan To LaneFollowing (PTLF)/InsideJudge1/If Action Subsystem/If Action Subsystem/Signal Latching/if action  ==
  In : Inport
  Action Port : ActionPort  ActionType=then
  Out : Outport
  wires:
  In/1 -> Out/1

== system LKAS_AutoSave_DF_20220315_0945/LKAS/LL/LLOn/LKA/Plan To LaneFollowing (PTLF)/InsideJudge1/If Action Subsystem/If Action Subsystem/Signal Latching1/if action  ==
  In : Inport
  Action Port : ActionPort  ActionType=then
  Out : Outport
  wires:
  In/1 -> Out/1

== system LKAS_AutoSave_DF_20220315_0945/LKAS/LL/LLOn/LKA/Plan To LaneFollowing (PTLF)/InsideJudge1/If Action Subsystem1/If Action Subsystem/Signal Latching/if action  ==
  In : Inport
  Action Port : ActionPort  ActionType=then
  Out : Outport
  wires:
  In/1 -> Out/1

== system LKAS_AutoSave_DF_20220315_0945/LKAS/LL/LLOn/LKA/Plan To LaneFollowing (PTLF)/InsideJudge1/If Action Subsystem1/If Action Subsystem/Signal Latching1/if action  ==
  In : Inport
  Action Port : ActionPort  ActionType=then
  Out : Outport
  wires:
  In/1 -> Out/1

== system LKAS_AutoSave_DF_20220315_0945/LKAS/LL/LLOn/LL State Determination (LLStateDet)/LL State Machine Conditions (LLSMCon)/Activation Condition (ActvC)/Deviation Threshold Condition (DvtThresCon)/Deviation Threshold Judgement LDW (DvtThresJdg)/Deviation Speed Detection (DvtSpdDet)/Ph1SWA ==
  Action Port : ActionPort  InitializeStates=reset  ActionType=then
      settings: AttributesFormatString=states = %<InitializeStates>
  Constant : Constant  OutDataTypeStr=single
  Out : Outport
      settings: AttributesFormatString=%<OutputWhenDisabled> = %<InitialOutput>
  wires:
  Constant/1 -> Out/1

== system LKAS_AutoSave_DF_20220315_0945/LKAS/LL/LLOn/LL State Determination (LLStateDet)/LL State Machine Conditions (LLSMCon)/Activation Condition (ActvC)/Deviation Threshold Condition (DvtThresCon)/Deviation Threshold Judgement LDW (DvtThresJdg)/Deviation Speed Detection (DvtSpdDet)/Ph2SWA ==
  Action Port : ActionPort  InitializeStates=reset  ActionType=elseif
      settings: AttributesFormatString=states = %<InitializeStates>
  Constant : Constant  Value=-1  OutDataTypeStr=single
  Out : Outport
      settings: AttributesFormatString=%<OutputWhenDisabled> = %<InitialOutput>
  wires:
  Constant/1 -> Out/1

== system LKAS_AutoSave_DF_20220315_0945/LKAS/LL/LLOn/LL State Determination (LLStateDet)/LL State Machine Conditions (LLSMCon)/Activation Condition (ActvC)/Deviation Threshold Condition (DvtThresCon)/Deviation Threshold Judgement LDW (DvtThresJdg)/Deviation Speed Detection (DvtSpdDet)/Ph3SWA ==
  In1 : Inport
  Action Port : ActionPort  InitializeStates=reset  ActionType=else
      settings: AttributesFormatString=states = %<InitializeStates>
  Out : Outport  OutDataTypeStr=single  InitialOutput=0
      settings: AttributesFormatString=%<OutputWhenDisabled> = %<InitialOutput>
  wires:
  In1/1 -> Out/1

== system LKAS_AutoSave_DF_20220315_0945/LKAS/LL/LLOn/LL State Determination (LLStateDet)/LL State Machine Conditions (LLSMCon)/Activation Condition (ActvC)/Deviation Threshold Condition (DvtThresCon)/Deviation Threshold Judgement LKA (DvtThresJdg)/Deviation Speed Detection (DvtSpdDet)/Ph1SWA ==
  Action Port : ActionPort  InitializeStates=reset  ActionType=then
      settings: AttributesFormatString=states = %<InitializeStates>
  Constant : Constant  OutDataTypeStr=single
  Out : Outport
      settings: AttributesFormatString=%<OutputWhenDisabled> = %<InitialOutput>
  wires:
  Constant/1 -> Out/1

== system LKAS_AutoSave_DF_20220315_0945/LKAS/LL/LLOn/LL State Determination (LLStateDet)/LL State Machine Conditions (LLSMCon)/Activation Condition (ActvC)/Deviation Threshold Condition (DvtThresCon)/Deviation Threshold Judgement LKA (DvtThresJdg)/Deviation Speed Detection (DvtSpdDet)/Ph2SWA ==
  Action Port : ActionPort  InitializeStates=reset  ActionType=elseif
      settings: AttributesFormatString=states = %<InitializeStates>
  Constant : Constant  Value=-1  OutDataTypeStr=single
  Out : Outport
      settings: AttributesFormatString=%<OutputWhenDisabled> = %<InitialOutput>
  wires:
  Constant/1 -> Out/1

== system LKAS_AutoSave_DF_20220315_0945/LKAS/LL/LLOn/LL State Determination (LLStateDet)/LL State Machine Conditions (LLSMCon)/Activation Condition (ActvC)/Deviation Threshold Condition (DvtThresCon)/Deviation Threshold Judgement LKA (DvtThresJdg)/Deviation Speed Detection (DvtSpdDet)/Ph3SWA ==
  Action Port : ActionPort  InitializeStates=reset  ActionType=else
      settings: AttributesFormatString=states = %<InitializeStates>
  Constant : Constant  Value=0  OutDataTypeStr=single
  Out : Outport
      settings: AttributesFormatString=%<OutputWhenDisabled> = %<InitialOutput>
  wires:
  Constant/1 -> Out/1

== system LKAS_AutoSave_DF_20220315_0945/LKAS/LL/LLOn/LL State Determination (LLStateDet)/LL State Machine Conditions (LLSMCon)/Deactivation Condition (DeactvC)/Deviation Threshold Condition (DvtThresCon)/Deviation Threshold Judgement LDW (DvtThresJdg)/Deviation Speed Detection (DvtSpdDet)/Ph1SWA ==
  Action Port : ActionPort  InitializeStates=reset  ActionType=then
      settings: AttributesFormatString=states = %<InitializeStates>
  Constant : Constant  OutDataTypeStr=single
  Out : Outport
      settings: AttributesFormatString=%<OutputWhenDisabled> = %<InitialOutput>
  wires:
  Constant/1 -> Out/1

== system LKAS_AutoSave_DF_20220315_0945/LKAS/LL/LLOn/LL State Determination (LLStateDet)/LL State Machine Conditions (LLSMCon)/Deactivation Condition (DeactvC)/Deviation Threshold Condition (DvtThresCon)/Deviation Threshold Judgement LDW (DvtThresJdg)/Deviation Speed Detection (DvtSpdDet)/Ph2SWA ==
  Action Port : ActionPort  InitializeStates=reset  ActionType=elseif
      settings: AttributesFormatString=states = %<InitializeStates>
  Constant : Constant  Value=-1  OutDataTypeStr=single
  Out : Outport
      settings: AttributesFormatString=%<OutputWhenDisabled> = %<InitialOutput>
  wires:
  Constant/1 -> Out/1

== system LKAS_AutoSave_DF_20220315_0945/LKAS/LL/LLOn/LL State Determination (LLStateDet)/LL State Machine Conditions (LLSMCon)/Deactivation Condition (DeactvC)/Deviation Threshold Condition (DvtThresCon)/Deviation Threshold Judgement LDW (DvtThresJdg)/Deviation Speed Detection (DvtSpdDet)/Ph3SWA ==
  In1 : Inport
  Action Port : ActionPort  InitializeStates=reset  ActionType=else
      settings: AttributesFormatString=states = %<InitializeStates>
  Out : Outport  OutDataTypeStr=single  InitialOutput=0
      settings: AttributesFormatString=%<OutputWhenDisabled> = %<InitialOutput>
  wires:
  In1/1 -> Out/1

== system LKAS_AutoSave_DF_20220315_0945/LKAS/LL/LLOn/LL State Determination (LLStateDet)/LL State Machine Conditions (LLSMCon)/Deactivation Condition (DeactvC)/Deviation Threshold Condition (DvtThresCon)/Deviation Threshold Judgement LDW (DvtThresJdg)/Deviation Threshold Condition Synthesis (DTCSyn)/Sum Condition ==
  In : Inport
  Sum : Inport  Port=2
  Enable : EnablePort  StatesWhenEnabling=reset
      settings: AttributesFormatString=states = %<StatesWhenEnabling>
  Add1 : Sum  OutDataTypeStr=single
  Memory : Memory  InheritSampleTime=on
  Relational Operator : RelationalOperator  Operator=<=  OutDataTypeStr=boolean  RndMeth=Nearest
  Saturation : Saturate  UpperLimit=5  LowerLimit=0
      settings: AttributesFormatString="Min = %<LowerLimit>  Max = %<UpperLimit>"
  Out : Outport  OutputWhenDisabled=reset  InitialOutput=0
      settings: AttributesFormatString=%<OutputWhenDisabled> = %<InitialOutput>
  wires:
  Relational Operator/1 -> Out/1
  Memory/1 -> Add1/2
  Add1/1 -> Saturation/1
  In/1 -> Add1/1
  Sum/1 -> Relational Operator/2
  Saturation/1 -> Memory/1, Relational Operator/1

== system LKAS_AutoSave_DF_20220315_0945/LKAS/LL/LLOn/LL State Determination (LLStateDet)/LL State Machine Conditions (LLSMCon)/Deactivation Condition (DeactvC)/Deviation Threshold Condition (DvtThresCon)/Deviation Threshold Judgement LKA (DvtThresJdg)/Deviation Speed Detection (DvtSpdDet)/Ph1SWA ==
  Action Port : ActionPort  InitializeStates=reset  ActionType=then
      settings: AttributesFormatString=states = %<InitializeStates>
  Constant : Constant  OutDataTypeStr=single
  Out : Outport
      settings: AttributesFormatString=%<OutputWhenDisabled> = %<InitialOutput>
  wires:
  Constant/1 -> Out/1

== system LKAS_AutoSave_DF_20220315_0945/LKAS/LL/LLOn/LL State Determination (LLStateDet)/LL State Machine Conditions (LLSMCon)/Deactivation Condition (DeactvC)/Deviation Threshold Condition (DvtThresCon)/Deviation Threshold Judgement LKA (DvtThresJdg)/Deviation Speed Detection (DvtSpdDet)/Ph2SWA ==
  Action Port : ActionPort  InitializeStates=reset  ActionType=elseif
      settings: AttributesFormatString=states = %<InitializeStates>
  Constant : Constant  Value=-1  OutDataTypeStr=single
  Out : Outport
      settings: AttributesFormatString=%<OutputWhenDisabled> = %<InitialOutput>
  wires:
  Constant/1 -> Out/1

== system LKAS_AutoSave_DF_20220315_0945/LKAS/LL/LLOn/LL State Determination (LLStateDet)/LL State Machine Conditions (LLSMCon)/Deactivation Condition (DeactvC)/Deviation Threshold Condition (DvtThresCon)/Deviation Threshold Judgement LKA (DvtThresJdg)/Deviation Speed Detection (DvtSpdDet)/Ph3SWA ==
  Action Port : ActionPort  InitializeStates=reset  ActionType=else
      settings: AttributesFormatString=states = %<InitializeStates>
  Constant : Constant  Value=0  OutDataTypeStr=single
  Out : Outport
      settings: AttributesFormatString=%<OutputWhenDisabled> = %<InitialOutput>
  wires:
  Constant/1 -> Out/1

== system LKAS_AutoSave_DF_20220315_0945/LKAS/LL/LLOn/LL State Determination (LLStateDet)/LL State Machine Conditions (LLSMCon)/Disable Condition (DisblC)/Driver Intent Condition (DrvInttC)/Take-Over Steering Check (TkOvStChk)/Time Delay (TDel)/If Action Subsystem ==
  Action Port : ActionPort  InitializeStates=reset  ActionType=then
      settings: AttributesFormatString=states = %<InitializeStates>
  Constant : Constant  OutDataTypeStr=boolean  SampleTime=-1
  Out : Outport
      settings: AttributesFormatString=%<OutputWhenDisabled> = %<InitialOutput>
  wires:
  Constant/1 -> Out/1

== system LKAS_AutoSave_DF_20220315_0945/LKAS/LL/LLOn/LL State Determination (LLStateDet)/LL State Machine Conditions (LLSMCon)/Disable Condition (DisblC)/Driver Intent Condition (DrvInttC)/Take-Over Steering Check (TkOvStChk)/Time Delay (TDel)/If Action Subsystem3 ==
  In1 : Inport
  Action Port : ActionPort  InitializeStates=reset  ActionType=else
      settings: AttributesFormatString=states = %<InitializeStates>
  Out : Outport
      settings: AttributesFormatString=%<OutputWhenDisabled> = %<InitialOutput>
  wires:
  In1/1 -> Out/1

== system LKAS_AutoSave_DF_20220315_0945/LKAS/LL/LLOn/LL State Determination (LLStateDet)/LL State Machine Conditions (LLSMCon)/Disable Condition (DisblC)/Driver Intent Condition (DrvInttC)/Take-Over Steering Check (TkOvStChk)/Time Delay (TDel)/Sum Condition1 ==
  SampleTime : Inport
  Sum : Inport  Port=2
  state = reset : EnablePort  StatesWhenEnabling=reset
  Add1 : Sum  OutDataTypeStr=single
  Memory : Memory  InheritSampleTime=on
  Relational Operator : RelationalOperator  Operator=<=  OutDataTypeStr=boolean  RndMeth=Nearest
  Saturation : Saturate  UpperLimit=10  LowerLimit=0
      settings: AttributesFormatString="Min = %<LowerLimit>  Max = %<UpperLimit>"
  Out : Outport  OutputWhenDisabled=reset  InitialOutput=0
      settings: AttributesFormatString=%<OutputWhenDisabled> = %<InitialOutput>
  wires:
  Memory/1 -> Add1/2
  Add1/1 -> Saturation/1
  SampleTime/1 -> Add1/1
  Sum/1 -> Relational Operator/2
  Relational Operator/1 -> Out/1
  Saturation/1 -> Memory/1, Relational Operator/1

== matlab function LKAS_AutoSave_DF_20220315_0945/LKAS/LL/Human Machine Interface (HMI)/HMI_Popup_Status ==
  data: HMI_Popup_Status output; stDACmode input; LKA_STATE input; HandsOff input; camera_common_fault input; Front_Camera_Blocked input; stFaultCSyn input
function HMI_Popup_Status = fcn(stDACmode,LKA_STATE,HandsOff,camera_common_fault,Front_Camera_Blocked,stFaultCSyn)
if stDACmode==2&&LKA_STATE==6 %车道保持辅助故障
    HMI_Popup_Status=uint8(6);
elseif stDACmode==2&&camera_common_fault==1&&Front_Camera_Blocked~=5  %车道保持辅助暂不可用
    HMI_Popup_Status=uint8(3);
elseif (stDACmode==2||stDACmode==1)&&(Front_Camera_Blocked==5)   %摄像头被遮挡
    HMI_Popup_Status=uint8(4);
elseif (stDACmode==2||stDACmode==1)&&HandsOff==1  %手握方向盘
    HMI_Popup_Status=uint8(2);    
elseif stDACmode==2&&(LKA_STATE==2)
    HMI_Popup_Status=uint8(1);
elseif stDACmode~=2&&stFaultCSyn==0
    HMI_Popup_Status=uint8(8);
elseif stFaultCSyn==0
    HMI_Popup_Status=uint8(7);
elseif stDACmode==2&&(LKA_STATE==0||LKA_STATE==1)
    HMI_Popup_Status=uint8(0);
else
    HMI_Popup_Status=uint8(0);
end

== matlab function LKAS_AutoSave_DF_20220315_0945/LKAS/LL/Human Machine Interface (HMI)/Hands_Off_Warning ==
  data: Hands_Off_Warning output; HandsOff input
function Hands_Off_Warning = fcn(HandsOff)
if HandsOff==0
    Hands_Off_Warning= uint8(0);
elseif HandsOff==1
    Hands_Off_Warning= uint8(1);
else
    Hands_Off_Warning= uint8(0);
end
